simulink model "PSC_tank_comunication"  (R2014a)
settings: Solver=ode1  StartTime=0.0  StopTime=inf  FixedStep=0.1  RelTol=1e-3
PostLoadFcn:
  | qc_set_target_type(getConfigSet(bdroot, 'QUARC Default Target Configuration'));
undefined symbols (not defined in the file or in its folder): HIL
libraries: quarc_library x3
settings Model: SimulationMode=external  ExtModeTrigDuration=30000  Creator=MLevis  LastModifiedBy=Aluno
settings SolverCC: PositivePriorityOrder=on
settings DataIOCC: SignalLoggingSaveFormat=ModelDataLogs
settings OptimizationCC: ExpressionDepthLimit=2147483647  InitFltsAndDblsToZero=on
settings DebuggingCC: SaveWithParameterizedLinksMsg=none  UnderspecifiedInitializationDetection=Classic  MultiTaskDSMMsg=warning  MultiTaskCondExecSysMsg=none  FcnCallInpInsideContextMsg=UseLocalSettings  StateNameClashWarn=warning
settings RTWCC: SystemTargetFile=quarc_win64.tlc  TemplateMakefile=quarc_default_tmf  Description=QUARC Win64 Target  ProcessScript=quarc_win64_make_rtw_hook
settings STFCustomTargetCC: CPPClassGenCompliant=on
settings GRTTargetCC: ParMdlRefBuildCompliant=off  CompOptLevelCompliant=off  CombineOutputUpdateFcns=off  MatFileLogging=off  GRTInterface=on  ExtMode=on  ExtModeMexFile=quarc_comm

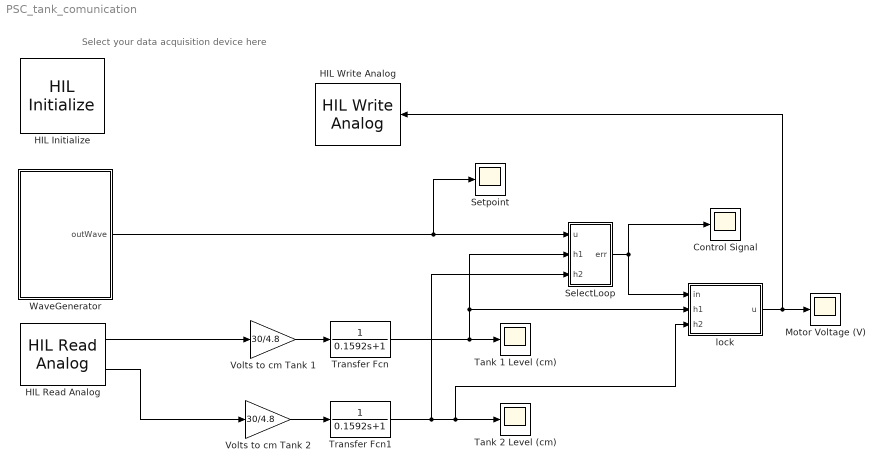
== system PSC_tank_comunication ==
  note: Select your data acquisition device here
  Control Signal : Scope
      settings: TimeRange=30  YMin=-30  YMax=30  SaveName=control_signal
  HIL Initialize : quarc_library/Data Acquisition/Generic/Configuration/HIL Initialize  object_name=HIL-1  board_type=q2_usb  board_number=0  board_options=d0=digital;d1=digital;led=auto;update_rate=normal;decimation=1  exclusive=off  active=off  hardware_clocks=[0]  clock_modes=[]  initial_clock_frequencies=[]  set_clock_params_at_start=off  set_clock_params_at_switch_in=off  set_clock_frequencies_at_start=off  set_clock_frequencies_at_switch_in=off  analog_input_channels=[0:1]  analog_input_maximums=10  analog_input_minimums=-10  set_analog_input_params_at_start=on  set_analog_input_params_at_switch_in=off  analog_output_channels=[0:1]  analog_output_maximums=10  analog_output_minimums=-10  initial_analog_outputs=[0]  final_analog_outputs=[0]  watchdog_analog_outputs=0  set_analog_output_params_at_start=on  set_analog_output_params_at_switch_in=off  set_analog_outputs_at_start=on  set_analog_outputs_at_switch_in=off  set_analog_outputs_at_terminate=on  set_analog_outputs_at_switch_out=off  set_analog_outputs_on_watchdog=off  digital_input_channels=[]  digital_output_channels=[]  digital_output_configuration=[]  initial_digital_outputs=[1]  final_digital_outputs=[1]  watchdog_digital_outputs=[1]  set_digital_output_params_at_start=off  set_digital_output_params_at_switch_in=off  set_digital_outputs_at_start=on  set_digital_outputs_at_switch_in=off  set_digital_outputs_at_terminate=on  set_digital_outputs_at_switch_out=off  set_digital_outputs_on_watchdog=off  encoder_channels=[0:1]  quadrature=[4]  encoder_filter_frequency=[]  initial_encoder_counts=[0]  set_encoder_params_at_start=on  set_encoder_params_at_switch_in=off  set_encoder_counts_at_start=on  set_encoder_counts_at_switch_in=off  pwm_channels=[]  pwm_modes=[0]  pwm_frequency=1/0.020  pwm_configuration=[]  pwm_alignment=[]  pwm_polarity=[]  pwm_leading_deadband=[]  pwm_trailing_deadband=[]  initial_pwm_outputs=[0]  final_pwm_outputs=[0]  watchdog_pwm_outputs=[0]  set_pwm_params_at_start=on  set_pwm_params_at_switch_in=off  set_pwm_outputs_at_start=on  set_pwm_outputs_at_switch_in=off  set_pwm_outputs_at_terminate=on  set_pwm_outputs_at_switch_out=off  set_pwm_outputs_on_watchdog=off  other_output_channels=[]  initial_other_outputs=[]  final_other_outputs=[]  watchdog_other_outputs=[]  set_other_outputs_at_start=off  set_other_outputs_at_switch_in=off  set_other_outputs_at_terminate=off  set_other_outputs_at_switch_out=off  set_other_outputs_on_watchdog=off
  HIL Read Analog : quarc_library/Data Acquisition/Generic/Immediate I//O/HIL Read Analog  object_name=HIL-1  channels=[0:1]  sample_time=qc_get_step_size  active=on  vector_output=off
  HIL Write Analog : quarc_library/Data Acquisition/Generic/Immediate I//O/HIL Write Analog  object_name=HIL-1  channels=0  sample_time=-1  active=off  vector_input=off
  Motor Voltage (V) : Scope
      settings: TimeRange=120  SaveName=motor_voltage
  SelectLoop : Subsystem
  Setpoint : Scope
      settings: TimeRange=30  YMin=-31  YMax=31  SaveName=setpoint
  Tank 1 Level (cm) : Scope
      settings: TickLabels=on  TimeRange=120  YMin=-2  YMax=30.5  SaveName=htank1
  Tank 2 Level (cm) : Scope
      settings: TimeRange=120  YMin=0  YMax=30  SaveName=htank2
  Transfer Fcn : TransferFcn  Denominator=[0.1592 1]
  Transfer Fcn1 : TransferFcn  Denominator=[0.1592 1]
  "Volts to cm Tank 1 " : Gain  Gain=30/4.8
  Volts to cm Tank 2 : Gain  Gain=30/4.8
  WaveGenerator : Subsystem
  lock : MATLAB Function  TreatAsAtomicUnit=on
  wires:
  HIL Read Analog/1 -> "Volts to cm Tank 1 "/1
  "Volts to cm Tank 1 "/1 -> Transfer Fcn/1
  Transfer Fcn1/1 -> SelectLoop/3(h2), lock/3(h2), Tank 2 Level (cm)/1
  Volts to cm Tank 2/1 -> Transfer Fcn1/1
  HIL Read Analog/2 -> Volts to cm Tank 2/1
  Transfer Fcn/1 -> lock/2(h1), SelectLoop/2(h1), Tank 1 Level (cm)/1
  WaveGenerator/1(outWave) -> Setpoint/1, SelectLoop/1(u)
  SelectLoop/1(err) -> Control Signal/1, lock/1(in)
  lock/1(u) -> Motor Voltage (V)/1, HIL Write Analog/1

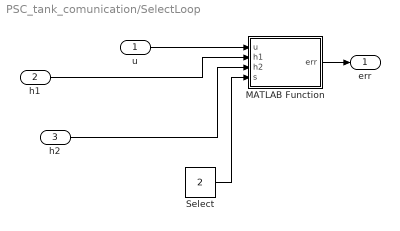
== system PSC_tank_comunication/SelectLoop ==
  u : Inport
  h1 : Inport  Port=2
  h2 : Inport  Port=3
  MATLAB Function : MATLAB Function  TreatAsAtomicUnit=on
  Select : Constant  Value=2
  err : Outport
  wires:
  u/1 -> MATLAB Function/1(u)
  Select/1 -> MATLAB Function/4(s)
  h1/1 -> MATLAB Function/2(h1)
  MATLAB Function/1(err) -> err/1
  h2/1 -> MATLAB Function/3(h2)

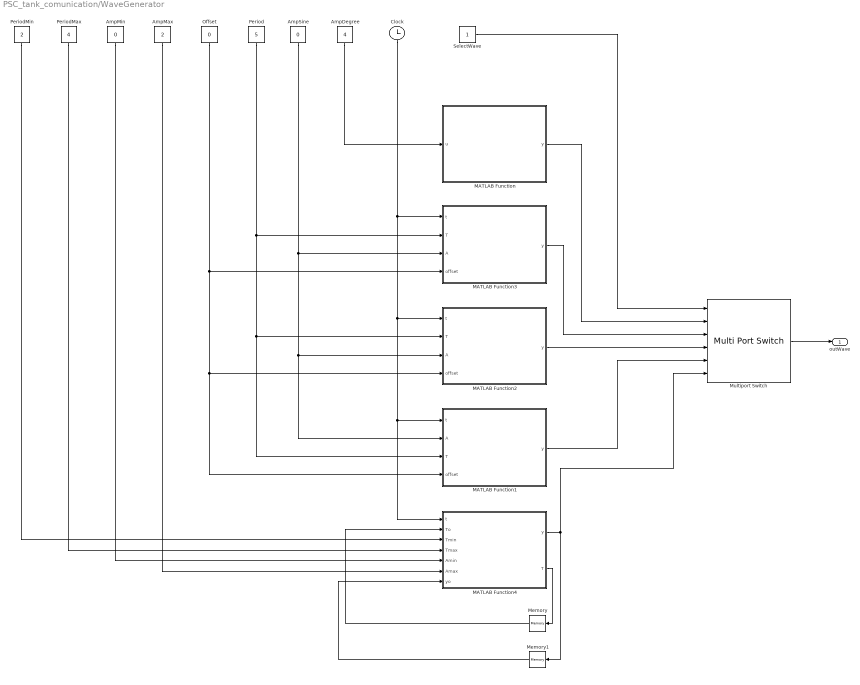
== system PSC_tank_comunication/WaveGenerator ==
  AmpDegree : Constant  Value=4
  AmpMax : Constant  Value=2
  AmpMin : Constant  Value=0
  AmpSine : Constant  Value=0
  Clock : Clock
  MATLAB Function : MATLAB Function  TreatAsAtomicUnit=on
  MATLAB Function1 : MATLAB Function  TreatAsAtomicUnit=on
  MATLAB Function2 : MATLAB Function  TreatAsAtomicUnit=on
  MATLAB Function3 : MATLAB Function  TreatAsAtomicUnit=on
  MATLAB Function4 : MATLAB Function  TreatAsAtomicUnit=on
  Memory : Memory
  Memory1 : Memory
  Multiport Switch : MultiPortSwitch  Inputs=5
  Offset : Constant  Value=0
  Period : Constant  Value=5
  PeriodMax : Constant  Value=4
  PeriodMin : Constant  Value=2
  SelectWave : Constant
  outWave : Outport
  wires:
  SelectWave/1 -> Multiport Switch/1
  Multiport Switch/1 -> outWave/1
  Clock/1 -> MATLAB Function2/1(t), MATLAB Function4/1(t), MATLAB Function1/1(t), MATLAB Function3/1(t)
  AmpSine/1 -> MATLAB Function3/3(A), MATLAB Function1/2(A), MATLAB Function2/3(A)
  Period/1 -> MATLAB Function3/2(T), MATLAB Function2/2(T), MATLAB Function1/3(T)
  Offset/1 -> MATLAB Function3/4(offset), MATLAB Function2/4(offset), MATLAB Function1/4(offset)
  AmpMax/1 -> MATLAB Function4/6(Amax)
  AmpMin/1 -> MATLAB Function4/5(Amin)
  PeriodMax/1 -> MATLAB Function4/4(Tmax)
  PeriodMin/1 -> MATLAB Function4/3(Tmin)
  MATLAB Function4/2(T) -> Memory/1
  MATLAB Function4/1(y) -> Memory1/1, Multiport Switch/6
  Memory/1 -> MATLAB Function4/2(To)
  Memory1/1 -> MATLAB Function4/7(yo)
  MATLAB Function/1(y) -> Multiport Switch/2
  MATLAB Function3/1(y) -> Multiport Switch/3
  MATLAB Function2/1(y) -> Multiport Switch/4
  MATLAB Function1/1(y) -> Multiport Switch/5
  AmpDegree/1 -> MATLAB Function/1(u)

== matlab function PSC_tank_comunication/WaveGenerator/MATLAB Function1 ==
  data: t input; A input; y output; T input; offset input
function y = sinusoidal_wave(t, A, T, offset)

y = A * sin( (1/T) * 2 * pi * t ) + offset;

== matlab function PSC_tank_comunication/WaveGenerator/MATLAB Function ==
  data: u input; y output
function y = degree_wave(u)
y = u;

== matlab function PSC_tank_comunication/WaveGenerator/MATLAB Function2 ==
  data: t input; y output; T input; A input; offset input
function y = square_wave(t, T, A, offset)
if( mod(t,T) < T/2 )
    y = A + offset;
else
    y = -A + offset;
end

== matlab function PSC_tank_comunication/WaveGenerator/MATLAB Function3 ==
  data: t input; y output; T input; A input; offset input
function y = sawtooth_wave(t, T, A, offset)
y = 2*( A * mod(t, T) ) / T + offset - A;

== matlab function PSC_tank_comunication/WaveGenerator/MATLAB Function4 ==
  data: t input; To input; y output; T output; Tmin input; Tmax input; Amin input; Amax input; yo input
function [y, T] = random_wave(t, To, Tmin, Tmax, Amin, Amax, yo)

in_rand_min = 0;
in_rand_max = 1;
out_T_min = Tmin;
out_T_max = Tmax;
out_A_min = Amin;
out_A_max = Amax;


if (t == 0)
    yo = 0;
    To = 0;
end

if ( To ~= 0 && t < To )
    y = yo;
    T = To;
else
    r1 = rand(1,1);
    r2 = rand(1,1);
    T = t + (r1 - in_rand_min) * (out_T_max - out_T_min) / (in_rand_max - in_rand_min) + out_T_min;
    y = (r2 - in_rand_min) * (out_A_max - out_A_min) / (in_rand_max - in_rand_min) + out_A_min;
end

== matlab function PSC_tank_comunication/lock ==
  data: in input; u output; h1 input; h2 input
function u = lock(in, h1, h2)

MAX_VOLTAGE = 4;
MAX_VOLTAGE_EXP = 3.2;
dh = 2.0;
setLimit = 30.2;

u = max(-MAX_VOLTAGE , in);
u = min(u , MAX_VOLTAGE);

if h2 + dh >= setLimit && h1 > dh && u >= 0
    u = -MAX_VOLTAGE;
end
if h1 + dh >= setLimit && u > 0
    u = MAX_VOLTAGE_EXP;
end
if h1 < dh && u < 0
    u = 0;
end

== matlab function PSC_tank_comunication/SelectLoop/MATLAB Function ==
  data: u input; err output; h1 input; h2 input; s input
function err = mux(u, h1, h2, s)
err = u;
if (s == 1)
    err = u - h1;
elseif (s == 2)
    err = u - h2;
end
